simulink model "sim_kalman_tune"  (R2024b)
settings: Solver=ode4  StartTime=t_0  StopTime=t_f  FixedStep=dt  RelTol=1e-8
settings Model: SimulationMode=accelerator  Creator=yevge  LastModifiedBy=Aiden Gaydos
settings DebuggingCC: AlgebraicLoopMsg=error  CheckMatrixSingularityMsg=error

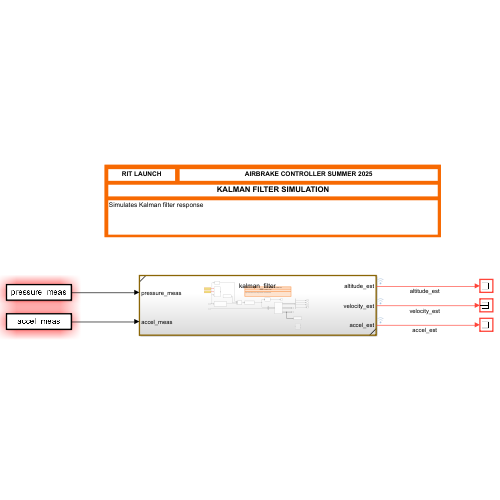
[thumbnail: Simulink's stored preview of the top-level diagram]
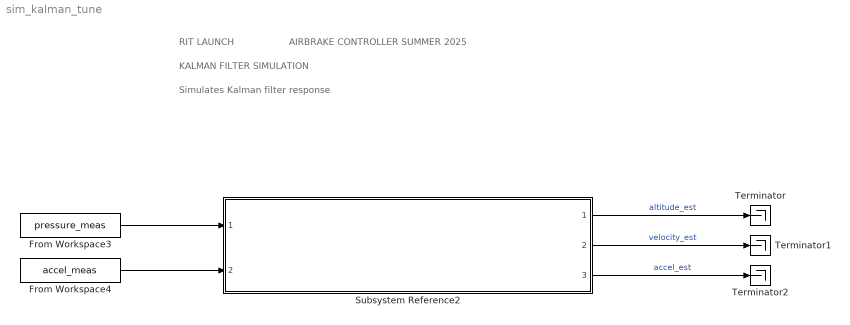
== system sim_kalman_tune ==
  note: AIRBRAKE CONTROLLER SUMMER 2025
  note: RIT LAUNCH
  note: KALMAN FILTER SIMULATION
  note: Simulates Kalman filter response
  From Workspace3 : FromWorkspace  VariableName=pressure_meas
  From Workspace4 : FromWorkspace  VariableName=accel_meas
  Subsystem Reference2 : Subsystem  ReferencedSubsystem=kalman_filter
  Terminator : Terminator
  Terminator1 : Terminator
  Terminator2 : Terminator
  wires:
  Subsystem Reference2/1 -> Terminator/1  "altitude_est"
  Subsystem Reference2/2 -> Terminator1/1  "velocity_est"
  Subsystem Reference2/3 -> Terminator2/1  "accel_est"
  From Workspace3/1 -> Subsystem Reference2/1
  From Workspace4/1 -> Subsystem Reference2/2
